simulink model "MainNew"  (R2021b)
settings: Solver=VariableStepAuto  StartTime=0.0  StopTime=10.0  RelTol=1e-3
undefined symbols (not defined in the file): c_Fuel, CM_FUEL_b, cmFuel_cmL, k_Fuel, L_TV, m_dot, m_iFuel, VRfromNED_cordT, W_LANDER
libraries: matrix_library x3, slpidlib x1, dspsrcs4 x1, shared6dof x1, aerolibanim x1, vrlib x1
settings Model: Creator=josepfamador  LastModifiedBy=josepfamador

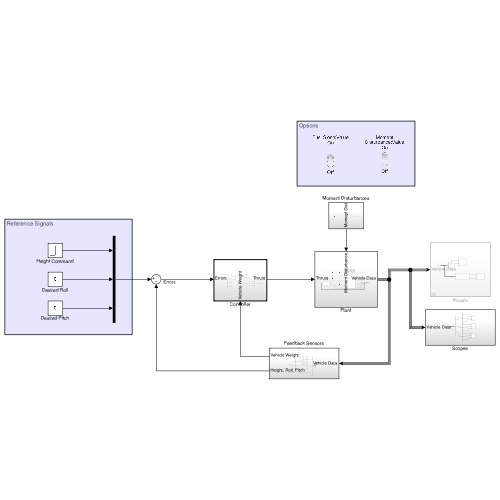
[thumbnail: Simulink's stored preview of the top-level diagram]
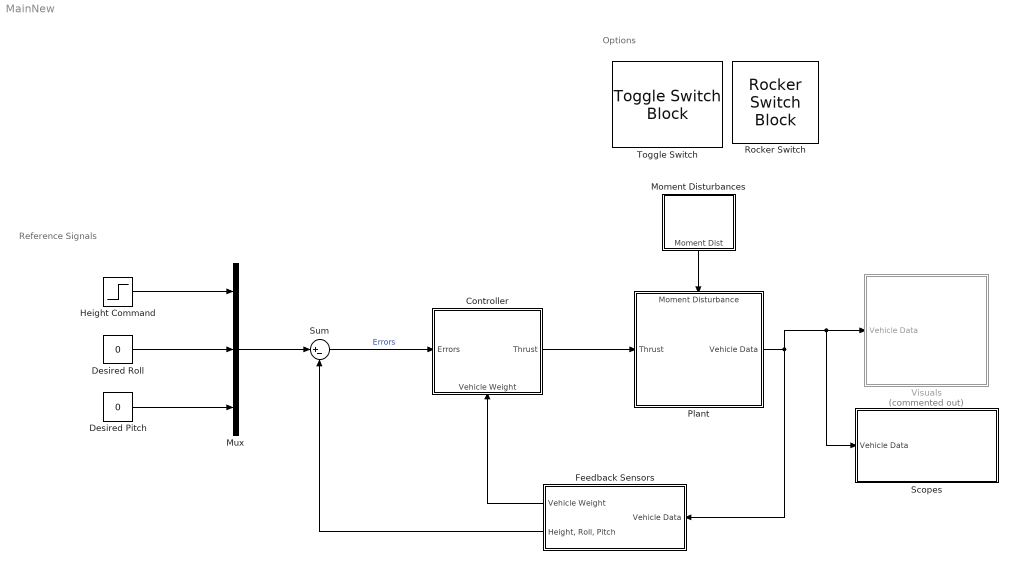
== system MainNew ==
  note: Options
  note: Reference Signals
  Controller : Subsystem  TreatAsAtomicUnit=on
      settings: PortSchema="{\"entries\":[{\"content\":{\"sides\":[{\"content\":{\"connectorIds\":[\"In1\"]},\"type\":\"ConnectorPlacement.EquallySpacedRectSide\",\"uuid\":\"a9e81047-82e7-465f-ace1-8f718b90561e\"},{\"content\":{\"connectorIds\":[\"Out1\"],\"side\":\"RIGHT\"},\"type\":\"ConnectorPlacement.EquallySpacedRectSide\",\"uuid\":\"e48627af-c2aa-4531-b804-41f44ff16765\"},{\"content\":{\"connectorIds\":[],\"side\":\"TOP\"},\"type\":\"ConnectorPlacement.EquallySpacedRectSide\",\"uuid\":\"f9e16229-b89b-4f8f-8331-a0f549979ea4\"},{\"content\":{\"connectorIds\":[\"In2\"],\"side\":\"BOTTOM\"},\"type\":\"ConnectorPlacement.EquallySpacedRectSide\",\"uuid\":\"04cdfde2-d4f0-49a2-8a73-ed462fcd7361\"}]},\"type\":\"ConnectorPlacement.EquallySpacedConnector\",\"uuid\":\"554d82b7-b70e-4d8b-909f-79f77f042d74\"}],\"packageUris\":[\"http://schema.mathworks.com/mf0/Connector/R2020b\"],\"version\":\"1.0\"}"
  Desired Pitch : Constant  Value=0
  Desired Roll : Constant  Value=0
  Feedback Sensors : Subsystem
  Height Command : Step  SampleTime=0
  Moment Disturbances : Subsystem
  Mux : Mux  Inputs=3
  Plant : Subsystem
      settings: PortSchema="{\"entries\":[{\"content\":{\"sides\":[{\"content\":{\"connectorIds\":[\"In1\"]},\"type\":\"ConnectorPlacement.EquallySpacedRectSide\",\"uuid\":\"a9e81047-82e7-465f-ace1-8f718b90561e\"},{\"content\":{\"connectorIds\":[\"Out1\"],\"side\":\"RIGHT\"},\"type\":\"ConnectorPlacement.EquallySpacedRectSide\",\"uuid\":\"e48627af-c2aa-4531-b804-41f44ff16765\"},{\"content\":{\"connectorIds\":[\"In2\"],\"side\":\"TOP\"},\"type\":\"ConnectorPlacement.EquallySpacedRectSide\",\"uuid\":\"f9e16229-b89b-4f8f-8331-a0f549979ea4\"}]},\"type\":\"ConnectorPlacement.EquallySpacedConnector\",\"uuid\":\"554d82b7-b70e-4d8b-909f-79f77f042d74\"}],\"packageUris\":[\"http://schema.mathworks.com/mf0/Connector/R2020b\"],\"version\":\"1.0\"}"
  Rocker Switch : RockerSwitchBlock
      settings: Values={{'Off', 'On'}, [0 1]}
  Scopes : Subsystem
  Sum : Sum  Inputs=|+-
  Toggle Switch : ToggleSwitchBlock
      settings: Values={{'Off', 'On'}, [0 1]}
  Visuals : Subsystem  Commented=on
  wires:
  Moment Disturbances/1(Moment Dist) -> Plant/2(Moment Disturbance)
  Plant/1(Vehicle Data) -> Feedback Sensors/1(Vehicle Data), Scopes/1(Vehicle Data), Visuals/1(Vehicle Data)
  Desired Pitch/1 -> Mux/3
  Desired Roll/1 -> Mux/2
  Height Command/1 -> Mux/1
  Mux/1 -> Sum/1
  Feedback Sensors/2("Height, Roll, Pitch") -> Sum/2
  Sum/1 -> Controller/1(Errors)  "Errors"
  Controller/1(Thrust) -> Plant/1(Thrust)
  Feedback Sensors/1(Vehicle Weight) -> Controller/2(Vehicle Weight)

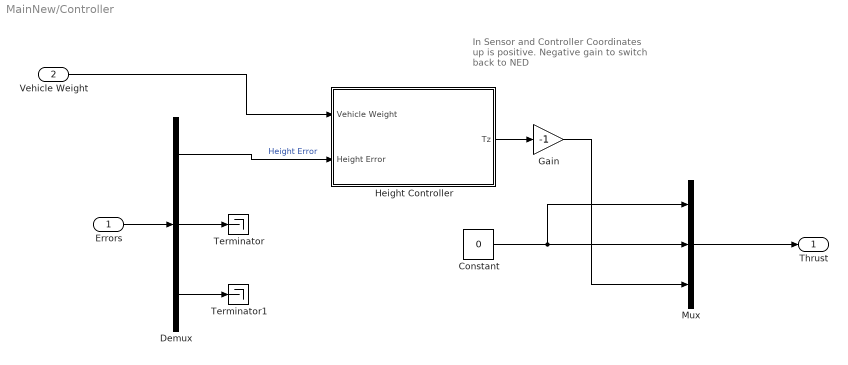
== system MainNew/Controller ==
  note: In Sensor and Controller Coordinates up is positive. Negative gain to switch back to NED
  Errors : Inport
  Vehicle Weight : Inport  Port=2
  Constant : Constant  Value=0
  Demux : Demux  Outputs=3
  Gain : Gain  Gain=-1
  Height Controller : Subsystem
  Mux : Mux  Inputs=3
  Terminator : Terminator
  Terminator1 : Terminator
  Thrust : Outport
  wires:
  Errors/1 -> Demux/1
  Demux/1 -> Height Controller/2(Height Error)  "Height Error"
  Vehicle Weight/1 -> Height Controller/1(Vehicle Weight)
  Mux/1 -> Thrust/1
  Height Controller/1(Tz) -> Gain/1
  Constant/1 -> Mux/2, Mux/1
  Demux/2 -> Terminator/1
  Demux/3 -> Terminator1/1
  Gain/1 -> Mux/3

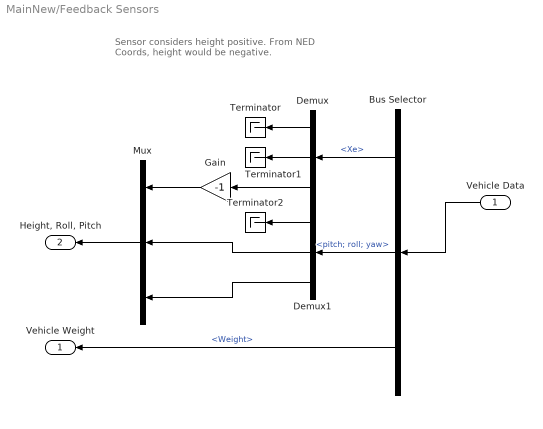
== system MainNew/Feedback Sensors ==
  note: Sensor considers height positive.
      | From NED Coords, height would be negative.
  Vehicle Data : Inport
  Bus Selector : BusSelector  OutputSignals=Xe,pitch; roll; yaw,Weight
  Demux : Demux  Outputs=3
  Demux1 : Demux  Outputs=3
  Gain : Gain  Gain=-1
  Mux : Mux  Inputs=3
  Terminator : Terminator
  Terminator1 : Terminator
  Terminator2 : Terminator
  Vehicle Weight : Outport
  "Height, Roll, Pitch" : Outport  Port=2
  wires:
  Vehicle Data/1 -> Bus Selector/1
  Bus Selector/1 -> Demux/1  "<Xe>"
  Bus Selector/2 -> Demux1/1  "<pitch; roll; yaw>"
  Demux/3 -> Gain/1
  Demux1/2 -> Mux/2
  Demux1/3 -> Mux/3
  Demux/1 -> Terminator/1
  Demux/2 -> Terminator1/1
  Demux1/1 -> Terminator2/1
  Mux/1 -> "Height, Roll, Pitch"/1
  Gain/1 -> Mux/1
  Bus Selector/3 -> Vehicle Weight/1  "<Weight>"

== system MainNew/Moment Disturbances ==
  Disturbance Vector : Subsystem
  Moment Disturbance : Constant  Value=0
  Slider : SliderBlock  ScaleMax=20
  Moment Dist : Outport
  wires:
  Disturbance Vector/1(Out1) -> Moment Dist/1
  Moment Disturbance/1 -> Disturbance Vector/Enable

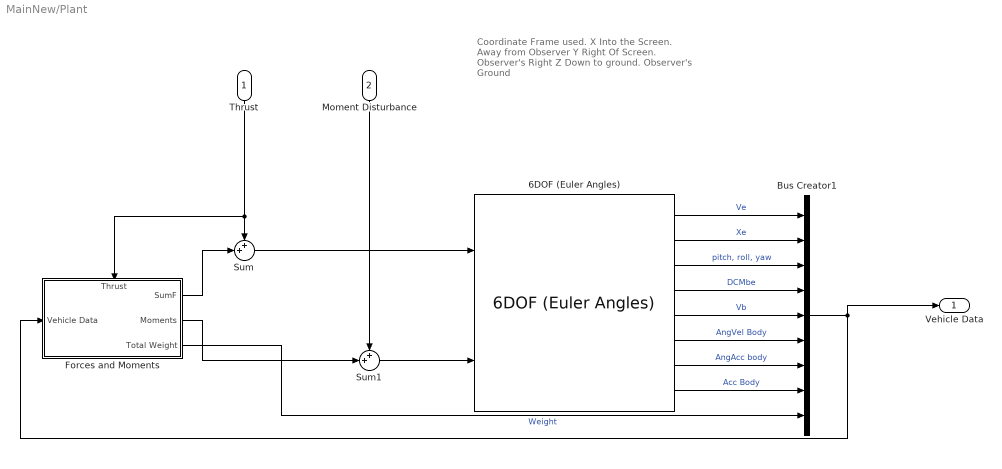
== system MainNew/Plant ==
  note: Coordinate Frame used.
      | X
      | Into the Screen. Away from Observer
      |
      | Y
      | Right Of Screen. Observer's Right
      |
      | Z
      | Down to ground. Observer's Ground
  Thrust : Inport
  Moment Disturbance : Inport  Port=2
  6DOF (Euler Angles) : shared6dof/6DOF (Euler Angles)  units=Metric (MKS)  mtype=Fixed  rep=Euler Angles  xme_0=[0 0 0]  Vm_0=[0 0 0]  eul_0=[0 0 0]  pm_0=[0 0 0]  mass_0=M_lander  mass_e=0.5  mass_f=2.0  inertia=I  inertia_e=eye(3)  inertia_f=2*eye(3)  k_quat=1.0  vre_flag=on  abi_flag=off  aMode=0  xme_statename=''  Vm_statename=''  eul_statename=''  quat_statename=''  pm_statename=''  mass_statename=''
      settings: SourceProductBaseCode=AE,PW,DR,MT,UV,VE
  Bus Creator1 : BusCreator  Inputs=9
  Forces and Moments : Subsystem
      settings: PortSchema="{\"entries\":[{\"content\":{\"sides\":[{\"content\":{\"connectorIds\":[\"In1\"]},\"type\":\"ConnectorPlacement.EquallySpacedRectSide\",\"uuid\":\"828f15e3-cbad-415f-85fb-ba6a8e0cd3b9\"},{\"content\":{\"connectorIds\":[\"Out1\",\"Out2\",\"Out3\"],\"side\":\"RIGHT\"},\"type\":\"ConnectorPlacement.EquallySpacedRectSide\",\"uuid\":\"5000816a-8e0b-4f65-bf77-7d05076903d9\"},{\"content\":{\"connectorIds\":[\"In2\"],\"side\":\"TOP\"},\"type\":\"ConnectorPlacement.EquallySpacedRectSide\",\"uuid\":\"57f53c13-0af9-4c97-9cf0-1ba4f356b699\"}]},\"type\":\"ConnectorPlacement.EquallySpacedConnector\",\"uuid\":\"7fdc047f-04f4-4b62-afef-380f9e9b929b\"}],\"packageUris\":[\"http://schema.mathworks.com/mf0/Connector/R2020b\"],\"version\":\"1.0\"}"
  Sum : Sum  Inputs=++|
  Sum1 : Sum  Inputs=++|
  Vehicle Data : Outport
  wires:
  6DOF (Euler Angles)/7 -> Bus Creator1/7  "AngAcc body"
  6DOF (Euler Angles)/3 -> Bus Creator1/3  "pitch, roll, yaw"
  Sum/1 -> 6DOF (Euler Angles)/1
  Thrust/1 -> Forces and Moments/2(Thrust), Sum/1
  6DOF (Euler Angles)/4 -> Bus Creator1/4  "DCMbe"
  Forces and Moments/1(SumF) -> Sum/2
  Forces and Moments/2(Moments) -> Sum1/2
  6DOF (Euler Angles)/6 -> Bus Creator1/6  "AngVel Body"
  6DOF (Euler Angles)/1 -> Bus Creator1/1  "Ve"
  6DOF (Euler Angles)/2 -> Bus Creator1/2  "Xe"
  6DOF (Euler Angles)/5 -> Bus Creator1/5  "Vb"
  6DOF (Euler Angles)/8 -> Bus Creator1/8  "Acc Body"
  Bus Creator1/1 -> Vehicle Data/1, Forces and Moments/1(Vehicle Data)
  Sum1/1 -> 6DOF (Euler Angles)/2
  Moment Disturbance/1 -> Sum1/1
  Forces and Moments/3(Total Weight) -> Bus Creator1/9  "Weight"

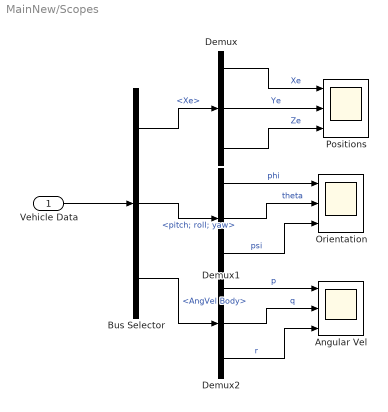
== system MainNew/Scopes ==
  Vehicle Data : Inport
  Angular Vel : Scope  NumInputPorts=3
  Bus Selector : BusSelector  OutputSignals=Xe,pitch; roll; yaw,AngVel Body
  Demux : Demux  Outputs=3
  Demux1 : Demux  Outputs=3
  Demux2 : Demux  Outputs=3
  Orientation : Scope  NumInputPorts=3
  Positions : Scope  NumInputPorts=3
  wires:
  Vehicle Data/1 -> Bus Selector/1
  Bus Selector/1 -> Demux/1  "<Xe>"
  Bus Selector/3 -> Demux2/1  "<AngVel Body>"
  Bus Selector/2 -> Demux1/1  "<pitch; roll; yaw>"
  Demux/2 -> Positions/2  "Ye"
  Demux/1 -> Positions/1  "Xe"
  Demux/3 -> Positions/3  "Ze"
  Demux1/1 -> Orientation/1  "phi"
  Demux1/2 -> Orientation/2  "theta"
  Demux1/3 -> Orientation/3  "psi"
  Demux2/2 -> Angular Vel/2  "q"
  Demux2/1 -> Angular Vel/1  "p"
  Demux2/3 -> Angular Vel/3  "r"

== system MainNew/Visuals ==
  Vehicle Data : Inport
  6DoF Animation1 : aerolibanim/6DoF Animation  u1=[-5 5 -5 5 0 4]  u2=0.1  u3=1  u4=[0 0 -1]  u5=Fixed position  u6=[-10 0 0]  u7=45  u8=off
  Bus Selector : BusSelector  OutputSignals=Xe,pitch; roll; yaw
  Coordinate Transforms : Subsystem
  VR Sink : vrlib/VR Sink  InstantiateOnLoad=on  SampleTime=0.1  ViewEnable=on  RemoteChange=off  RemoteView=off  FieldsWritten=Lander.rotation.4.1.1.double#Lander.translation.3.1.1.double  WorldFileName=/Users/josepfamador/RPL_controls/vrsinkstuff/V6b.x3d  AutoView=off  VideoDimensions=[]  AllowVariableSize=off
  wires:
  Bus Selector/1 -> 6DoF Animation1/1  "<Xe>"
  Bus Selector/2 -> 6DoF Animation1/2  "<pitch; roll; yaw>"
  Vehicle Data/1 -> Bus Selector/1, Coordinate Transforms/1(Vehicle Data)
  Coordinate Transforms/1(VR Rotation) -> VR Sink/1
  Coordinate Transforms/2(VR Translation) -> VR Sink/2

== system MainNew/Controller/Height Controller ==
  Vehicle Weight : Inport
  Height Error : Inport  Port=2
  Dot Product : DotProduct  InputSameDT=on  OutDataTypeStr=Inherit: Inherit via internal rule
  PID Controller : slpidlib/PID Controller  Controller=PID  Form=Parallel  TimeDomain=Continuous-time  UseExternalTs=off  SampleTime=-1  IntegratorMethod=Forward Euler  FilterMethod=Forward Euler  ControllerParametersSource=internal  P=0.203941393902336  I=0.000548507911387826  D=13.3428538970744  UseFilter=on  N=45.4968011971303  TunerSelectOption=Transfer Function Based (PID Tuner App)  InitialConditionSource=internal  InitialConditionForIntegrator=0  InitialConditionForFilter=0  DifferentiatorICPrevScaledInput=0  ExternalReset=none  TrackingMode=off  Kt=1  LimitOutput=off  SatLimitsSource=internal  UpperSaturationLimit=inf  LowerSaturationLimit=-inf  LinearizeAsGain=on  AntiWindupMode=none  Kb=1  POutMin=[]  POutMax=[]  IOutMin=[]  IOutMax=[]  DOutMin=[]  DOutMax=[]  NOutMin=[]  NOutMax=[]  SumOutMin=[]  SumOutMax=[]  SaturationOutMin=[]  SaturationOutMax=[]  PParamMin=[]  PParamMax=[]  IParamMin=[]  IParamMax=[]  DParamMin=[]  DParamMax=[]  NParamMin=[]  NParamMax=[]  KbParamMin=[]  KbParamMax=[]  KtParamMin=[]  KtParamMax=[]  KbOutMin=[]  KbOutMax=[]  KtOutMin=[]  KtOutMax=[]  IntegratorOutMin=[]  IntegratorOutMax=[]  FilterOutMin=[]  FilterOutMax=[]  SumI1OutMin=[]  SumI1OutMax=[]  SumI2OutMin=[]  SumI2OutMax=[]  SumI3OutMin=[]  SumI3OutMax=[]  SumI4OutMin=[]  SumI4OutMax=[]  SumDOutMin=[]  SumDOutMax=[]  DifferentiatorOutMin=[]  DifferentiatorOutMax=[]  FilterDiffOutCoefMin=[]  FilterDiffOutCoefMax=[]  ReciprocalOutMin=[]  ReciprocalOutMax=[]  SumDenOutMin=[]  SumDenOutMax=[]  SumNumOutMin=[]  SumNumOutMax=[]  DivideOutMin=[]  DivideOutMax=[]  UdiffTsProdOutMin=[]  UdiffTsProdOutMax=[]  NTsProdOutMin=[]  NTsProdOutMax=[]  UintegralTsProdOutMin=[]  UintegralTsProdOutMax=[]  UngainTsProdOutMin=[]  UngainTsProdOutMax=[]  IntegratorContinuousStateAttributes=''  IntegratorStateMustResolveToSignalObject=off  IntegratorRTWStateStorageClass=Auto  FilterContinuousStateAttributes=''  FilterStateMustResolveToSignalObject=off  FilterRTWStateStorageClass=Auto  ParallelPVariant=InternalParameters  IdealPVariant=Disabled  IVariant=InternalParameters  DVariant=InternalParameters  IntegratorVariant=Continuous  SatVariant=Disabled  AWVariant=Passthrough  PCopyVariant=Disabled  TRVariant=Disabled  FdbkBlocksVariant=Forward  IdealPFdbkVariant=Disabled  SatFdbkVariant=Disabled  DerivativeFilterVariant=ContFilter  NVariant=InternalParameters  NCopyVariant=Disabled  FilterICVariant=InternalICsFilter  IntegratorICVariant=InternalICs  ExternalResetVariant=Disabled  TRSumVariant=Passthrough  SumFdbkVariant=Disabled  SumVariant=Sum_PID  TsampFilterVariant=InternalTs  TsampNgainVariant=Passthrough  TsampIntegralVariant=Passthrough  ExternalSaturationOutDataTypeStr=Inherit: Same as second input
  Square Root : Sqrt  SaturateOnIntegerOverflow=on
  Sum : Sum  Inputs=++|
  Tz : Outport
  wires:
  Height Error/1 -> PID Controller/1
  Vehicle Weight/1 -> Dot Product/1, Dot Product/2
  Dot Product/1 -> Square Root/1
  PID Controller/1 -> Sum/2  "Thrust Difference"
  Square Root/1 -> Sum/1
  Sum/1 -> Tz/1

== system MainNew/Moment Disturbances/Disturbance Vector ==
  Enable : EnablePort
  Constant : Constant  Value=0
  Discrete Impulse : dspsrcs4/Discrete  Impulse  Delay=0  SampleTime=1  FrameSample=1  OutputFrames=off  dataType=double  isSigned=on  wordLen=16  udDataType=sfix(16)  fracBitsMode=Best precision  numFracBits=15  OutDataTypeStr=double  LastOutDataTypeStr=double
  Impulse Magnitude (Newtons) : Gain  Gain=0.3610372340425532
  Mux : Mux  Inputs=3
  Out1 : Outport
  wires:
  Mux/1 -> Out1/1
  Impulse Magnitude (Newtons)/1 -> Mux/2
  Discrete Impulse/1 -> Impulse Magnitude (Newtons)/1
  Constant/1 -> Mux/3, Mux/1

== system MainNew/Plant/Forces and Moments ==
  Vehicle Data : Inport
  Thrust : Inport  Port=2
  Forces Body Fixed Frame : Subsystem  TreatAsAtomicUnit=on
      settings: PortSchema="{\"entries\":[{\"content\":{\"sides\":[{\"content\":{\"connectorIds\":[\"In1\"]},\"type\":\"ConnectorPlacement.EquallySpacedRectSide\",\"uuid\":\"828f15e3-cbad-415f-85fb-ba6a8e0cd3b9\"},{\"content\":{\"connectorIds\":[\"Out1\",\"Out2\"],\"side\":\"RIGHT\"},\"type\":\"ConnectorPlacement.EquallySpacedRectSide\",\"uuid\":\"5000816a-8e0b-4f65-bf77-7d05076903d9\"},{\"content\":{\"connectorIds\":[],\"side\":\"TOP\"},\"type\":\"ConnectorPlacement.EquallySpacedRectSide\",\"uuid\":\"57f53c13-0af9-4c97-9cf0-1ba4f356b699\"},{\"content\":{\"connectorIds\":[\"Out3\",\"Out4\"],\"side\":\"BOTTOM\"},\"type\":\"ConnectorPlacement.EquallySpacedRectSide\",\"uuid\":\"07d00598-10e4-47df-ac26-33e6f3a9eead\"}]},\"type\":\"ConnectorPlacement.EquallySpacedConnector\",\"uuid\":\"7fdc047f-04f4-4b62-afef-380f9e9b929b\"}],\"packageUris\":[\"http://schema.mathworks.com/mf0/Connector/R2020b\"],\"version\":\"1.0\"}"
  Moments Body Fixed : Subsystem
      settings: PortSchema="{\"entries\":[{\"content\":{\"sides\":[{\"content\":{\"connectorIds\":[\"In1\"]},\"type\":\"ConnectorPlacement.EquallySpacedRectSide\",\"uuid\":\"bf632890-9061-4ebf-b839-17051433f7d2\"},{\"content\":{\"connectorIds\":[\"Out1\"],\"side\":\"RIGHT\"},\"type\":\"ConnectorPlacement.EquallySpacedRectSide\",\"uuid\":\"d3255547-983f-46fe-8ffa-de3f6c331a2a\"},{\"content\":{\"connectorIds\":[\"In2\",\"In3\"],\"side\":\"TOP\"},\"type\":\"ConnectorPlacement.EquallySpacedRectSide\",\"uuid\":\"18f3806f-6d56-407f-aadd-d25baf8c86b7\"}]},\"type\":\"ConnectorPlacement.EquallySpacedConnector\",\"uuid\":\"1b0eb8e4-97ea-4203-914f-8b852a07c841\"}],\"packageUris\":[\"http://schema.mathworks.com/mf0/Connector/R2020b\"],\"version\":\"1.0\"}"
  SumF : Outport
  Moments : Outport  Port=2
  Total Weight : Outport  Port=3
  wires:
  Forces Body Fixed Frame/1(SumF) -> SumF/1
  Moments Body Fixed/1(Moment) -> Moments/1
  Forces Body Fixed Frame/3(Fuel Slosh Vector) -> Moments Body Fixed/2(Slosh)
  Thrust/1 -> Moments Body Fixed/1(Thrust)
  Forces Body Fixed Frame/4(Weight Fuel (Body Fixed)) -> Moments Body Fixed/3(Weight Body Fixed)
  Vehicle Data/1 -> Forces Body Fixed Frame/1(Vehicle Data)
  Forces Body Fixed Frame/2(Total Weight) -> Total Weight/1

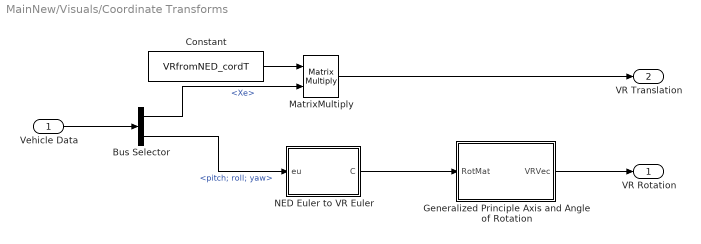
== system MainNew/Visuals/Coordinate Transforms ==
  Vehicle Data : Inport
  Bus Selector : BusSelector  OutputSignals=Xe,pitch; roll; yaw
  Constant : Constant  Value=VRfromNED_cordT
  Generalized Principle Axis and Angle of Rotation : MATLAB Function  TreatAsAtomicUnit=on
  MatrixMultiply : Product  Multiplication=Matrix(*)
  NED Euler to VR Euler : MATLAB Function  TreatAsAtomicUnit=on
  VR Rotation : Outport
  VR Translation : Outport  Port=2
  wires:
  Vehicle Data/1 -> Bus Selector/1
  Constant/1 -> MatrixMultiply/1
  Bus Selector/1 -> MatrixMultiply/2  "<Xe>"
  Bus Selector/2 -> NED Euler to VR Euler/1(eu)  "<pitch; roll; yaw>"
  NED Euler to VR Euler/1(C) -> Generalized Principle Axis and Angle of Rotation/1(RotMat)
  MatrixMultiply/1 -> VR Translation/1
  Generalized Principle Axis and Angle of Rotation/1(VRVec) -> VR Rotation/1

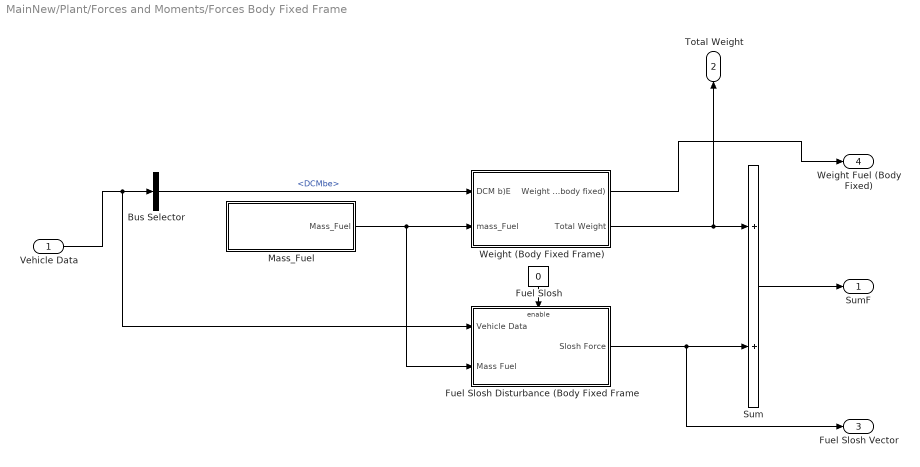
== system MainNew/Plant/Forces and Moments/Forces Body Fixed Frame ==
  Vehicle Data : Inport
  Bus Selector : BusSelector  OutputSignals=DCMbe
  Fuel Slosh : Constant  Value=0
  Fuel Slosh Disturbance (Body Fixed Frame : Subsystem
  Mass_Fuel : Subsystem
  Sum : Sum
  Weight (Body Fixed Frame) : Subsystem
  SumF : Outport
  Total Weight : Outport  Port=2
  Fuel Slosh Vector : Outport  Port=3
  Weight Fuel (Body Fixed) : Outport  Port=4
  wires:
  Mass_Fuel/1(Mass_Fuel) -> Fuel Slosh Disturbance (Body Fixed Frame/2(Mass Fuel), Weight (Body Fixed Frame)/2(mass_Fuel)
  Weight (Body Fixed Frame)/2(Total Weight) -> Total Weight/1, Sum/1
  Fuel Slosh Disturbance (Body Fixed Frame/1(Slosh Force) -> Fuel Slosh Vector/1, Sum/2
  Sum/1 -> SumF/1
  Fuel Slosh/1 -> Fuel Slosh Disturbance (Body Fixed Frame/Enable
  Weight (Body Fixed Frame)/1(Weight Fuel (body fixed)) -> Weight Fuel (Body Fixed)/1
  Vehicle Data/1 -> Fuel Slosh Disturbance (Body Fixed Frame/1(Vehicle Data), Bus Selector/1
  Bus Selector/1 -> Weight (Body Fixed Frame)/1(DCM b)E)  "<DCMbe>"

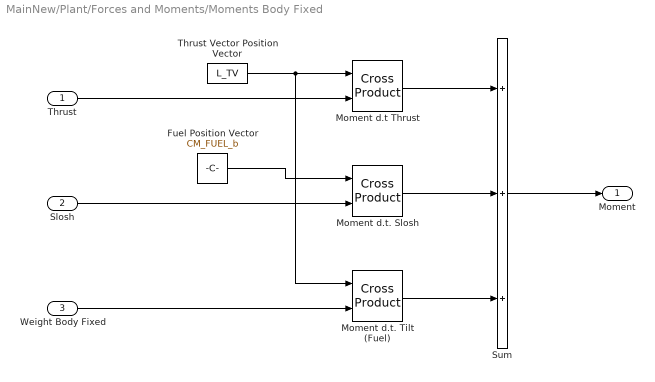
== system MainNew/Plant/Forces and Moments/Moments Body Fixed ==
  Thrust : Inport
  Slosh : Inport  Port=2
  Weight Body Fixed : Inport  Port=3
  Fuel Position Vector : Constant  Value=CM_FUEL_b
  Moment d.t Thrust : matrix_library/Cross Product
      settings: SourceProductBaseCode=SL
  Moment d.t. Slosh : matrix_library/Cross Product
      settings: SourceProductBaseCode=SL
  Moment d.t. Tilt (Fuel) : matrix_library/Cross Product
      settings: SourceProductBaseCode=SL
  Sum : Sum  Inputs=+++
  Thrust Vector Position Vector : Constant  Value=L_TV
  Moment : Outport
  wires:
  Thrust/1 -> Moment d.t Thrust/2
  Thrust Vector Position Vector/1 -> Moment d.t. Tilt (Fuel)/1, Moment d.t Thrust/1
  Slosh/1 -> Moment d.t. Slosh/2
  Fuel Position Vector/1 -> Moment d.t. Slosh/1
  Weight Body Fixed/1 -> Moment d.t. Tilt (Fuel)/2
  Moment d.t. Tilt (Fuel)/1 -> Sum/3
  Moment d.t. Slosh/1 -> Sum/2
  Moment d.t Thrust/1 -> Sum/1
  Sum/1 -> Moment/1

== system MainNew/Plant/Forces and Moments/Forces Body Fixed Frame/Fuel Slosh Disturbance (Body Fixed Frame ==
  note: 0 Disturbance in Z Body fixed Frame From Fuel Slosh
  Vehicle Data : Inport
  Mass Fuel : Inport  Port=2
  Enable : EnablePort
  Constant : Constant  Value=0
  Forces Slosh : Subsystem
  Mux : Mux  Inputs=3
  Subsystem : Subsystem
  Slosh Force : Outport
  wires:
  Subsystem/1("phi, phi_d, phi_dd") -> Forces Slosh/1("EA, EAd, EAdd")
  Subsystem/2("theta, theta_d, theta_dd") -> Forces Slosh/2("EA, EAd, EAdd1")
  Mass Fuel/1 -> Forces Slosh/3(Mass Fuel)
  Constant/1 -> Mux/3
  Forces Slosh/1(Fx) -> Mux/1
  Forces Slosh/2(Fy) -> Mux/2
  Mux/1 -> Slosh Force/1
  Vehicle Data/1 -> Subsystem/1(Vehicle Data)

== system MainNew/Plant/Forces and Moments/Forces Body Fixed Frame/Mass_Fuel ==
  note: m_dot set to 0
  Clock : Clock
  Sum : Sum  Inputs=+-|
  mass_burn_rate : Gain  Gain=m_dot
  mass_intial_fuel : Constant  Value=m_iFuel
  Mass_Fuel : Outport
  wires:
  mass_burn_rate/1 -> Sum/2
  Sum/1 -> Mass_Fuel/1
  mass_intial_fuel/1 -> Sum/1
  Clock/1 -> mass_burn_rate/1

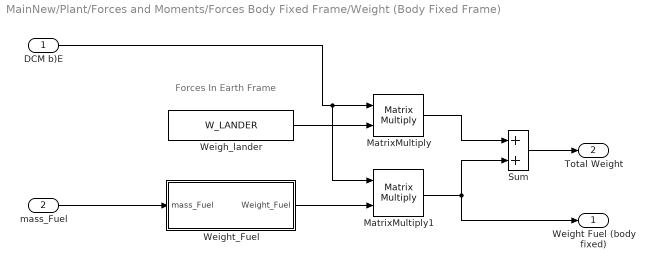
== system MainNew/Plant/Forces and Moments/Forces Body Fixed Frame/Weight (Body Fixed Frame) ==
  note: Forces In Earth Frame
  DCM b)E : Inport
  mass_Fuel : Inport  Port=2
  MatrixMultiply : Product  Multiplication=Matrix(*)
  MatrixMultiply1 : Product  Multiplication=Matrix(*)
  Sum : Sum
  Weigh_lander : Constant  Value=W_LANDER
  Weight_Fuel : Subsystem  TreatAsAtomicUnit=on
  Weight Fuel (body fixed) : Outport
  Total Weight : Outport  Port=2
  wires:
  mass_Fuel/1 -> Weight_Fuel/1(mass_Fuel)
  DCM b)E/1 -> MatrixMultiply1/1, MatrixMultiply/1
  MatrixMultiply1/1 -> Weight Fuel (body fixed)/1, Sum/2
  MatrixMultiply/1 -> Sum/1
  Weight_Fuel/1(Weight_Fuel) -> MatrixMultiply1/2
  Weigh_lander/1 -> MatrixMultiply/2
  Sum/1 -> Total Weight/1

== system MainNew/Plant/Forces and Moments/Forces Body Fixed Frame/Fuel Slosh Disturbance (Body Fixed Frame/Forces Slosh ==
  "EA, EAd, EAdd" : Inport
  "EA, EAd, EAdd1" : Inport  Port=2
  Mass Fuel : Inport  Port=3
  Constant : Constant  Value=cmFuel_cmL
  Subsystem1 : Subsystem
  Subsystem2 : Subsystem
  Fx : Outport
  Fy : Outport  Port=2
  wires:
  "EA, EAd, EAdd1"/1 -> Subsystem2/1("EA, EAd, EAdd")  "Pitch"
  Subsystem2/1(Fy) -> Fy/1
  "EA, EAd, EAdd"/1 -> Subsystem1/1("EA, EAd, EAdd")  "Roll"
  Subsystem1/1(Fx) -> Fx/1
  Constant/1 -> Subsystem2/3(Arm Length), Subsystem1/3(Arm Length)
  Mass Fuel/1 -> Subsystem1/2(Mass Fuel), Subsystem2/2(Mass Fuel)

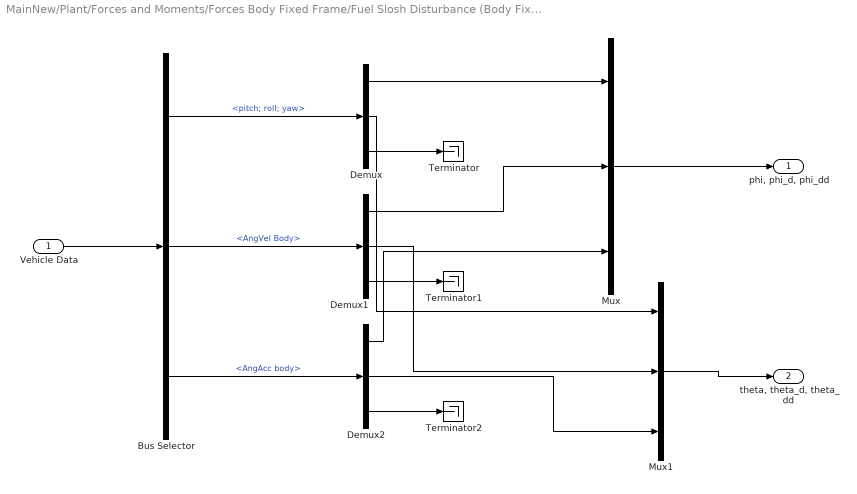
== system MainNew/Plant/Forces and Moments/Forces Body Fixed Frame/Fuel Slosh Disturbance (Body Fixed Frame/Subsystem ==
  Vehicle Data : Inport
  Bus Selector : BusSelector  OutputSignals=pitch; roll; yaw,AngVel Body,AngAcc body
  Demux : Demux  Outputs=3
  Demux1 : Demux  Outputs=3
  Demux2 : Demux  Outputs=3
  Mux : Mux  Inputs=3
  Mux1 : Mux  Inputs=3
  Terminator : Terminator
  Terminator1 : Terminator
  Terminator2 : Terminator
  "phi, phi_d, phi_dd" : Outport
  "theta, theta_d, theta_dd" : Outport  Port=2
  wires:
  Bus Selector/1 -> Demux/1  "<pitch; roll; yaw>"
  Bus Selector/2 -> Demux1/1  "<AngVel Body>"
  Bus Selector/3 -> Demux2/1  "<AngAcc body>"
  Demux/1 -> Mux/1
  Demux1/1 -> Mux/2
  Demux2/1 -> Mux/3
  Mux/1 -> "phi, phi_d, phi_dd"/1
  Demux/2 -> Mux1/1
  Demux1/2 -> Mux1/2
  Demux2/2 -> Mux1/3
  Demux/3 -> Terminator/1
  Demux1/3 -> Terminator1/1
  Demux2/3 -> Terminator2/1
  Mux1/1 -> "theta, theta_d, theta_dd"/1
  Vehicle Data/1 -> Bus Selector/1

== system MainNew/Plant/Forces and Moments/Forces Body Fixed Frame/Weight (Body Fixed Frame)/Weight_Fuel ==
  mass_Fuel : Inport
  Constant : Constant  Value=0
  Mux : Mux  Inputs=3
  Weight_Fuel : Outport
  wires:
  Constant/1 -> Mux/2, Mux/1
  mass_Fuel/1 -> Mux/3
  Mux/1 -> Weight_Fuel/1

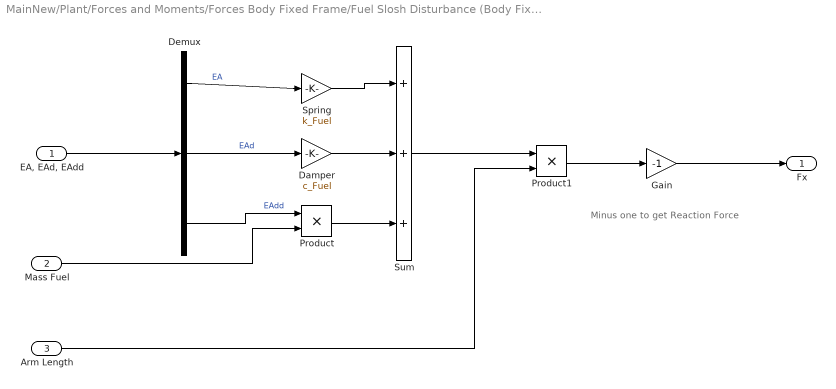
== system MainNew/Plant/Forces and Moments/Forces Body Fixed Frame/Fuel Slosh Disturbance (Body Fixed Frame/Forces Slosh/Subsystem1 ==
  note: Minus one to get Reaction Force
  "EA, EAd, EAdd" : Inport
  Mass Fuel : Inport  Port=2
  Arm Length : Inport  Port=3
  Damper : Gain  Gain=c_Fuel
  Demux : Demux  Outputs=3
  Gain : Gain  Gain=-1
  Product : Product
  Product1 : Product
  Spring : Gain  Gain=k_Fuel
  Sum : Sum  Inputs=+++
  Fx : Outport
  wires:
  Demux/1 -> Spring/1  "EA"
  Demux/2 -> Damper/1  "EAd"
  Demux/3 -> Product/1  "EAdd"
  Mass Fuel/1 -> Product/2
  Product/1 -> Sum/3
  Damper/1 -> Sum/2
  Spring/1 -> Sum/1
  "EA, EAd, EAdd"/1 -> Demux/1
  Sum/1 -> Product1/1
  Arm Length/1 -> Product1/2
  Product1/1 -> Gain/1
  Gain/1 -> Fx/1

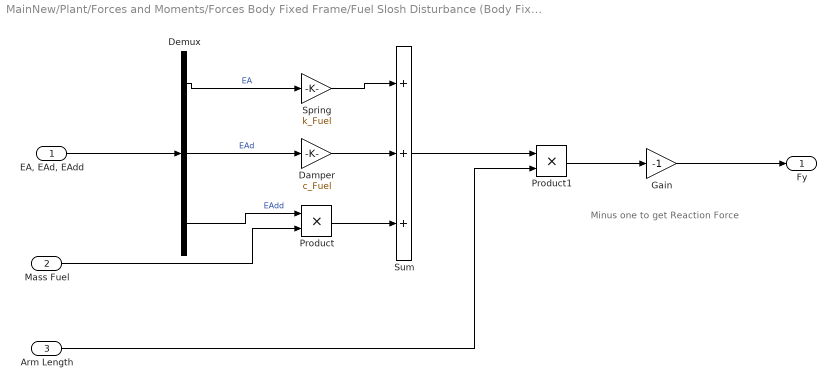
== system MainNew/Plant/Forces and Moments/Forces Body Fixed Frame/Fuel Slosh Disturbance (Body Fixed Frame/Forces Slosh/Subsystem2 ==
  note: Minus one to get Reaction Force
  "EA, EAd, EAdd" : Inport
  Mass Fuel : Inport  Port=2
  Arm Length : Inport  Port=3
  Damper : Gain  Gain=c_Fuel
  Demux : Demux  Outputs=3
  Gain : Gain  Gain=-1
  Product : Product
  Product1 : Product
  Spring : Gain  Gain=k_Fuel
  Sum : Sum  Inputs=+++
  Fy : Outport
  wires:
  Demux/1 -> Spring/1  "EA"
  Demux/2 -> Damper/1  "EAd"
  Demux/3 -> Product/1  "EAdd"
  Mass Fuel/1 -> Product/2
  Product/1 -> Sum/3
  Damper/1 -> Sum/2
  Spring/1 -> Sum/1
  "EA, EAd, EAdd"/1 -> Demux/1
  Sum/1 -> Product1/1
  Arm Length/1 -> Product1/2
  Product1/1 -> Gain/1
  Gain/1 -> Fy/1

== matlab function MainNew/Visuals/Coordinate Transforms/Generalized Principle Axis and Angle of Rotation ==
  data: VRVec output; RotMat input
function VRVec  = fcn(RotMat)
% Rotation algorithms obtained form "Spacecraft Dynamics & Control (ARO
% 4090 text) pg 21 
phi = acos((trace(RotMat) -  1)/2); % eq 1.27
A = 1/(sin(phi)) * [RotMat(2,3) - RotMat(3,2)
                    RotMat(3,1) - RotMat(1,3)
                    RotMat(1,2) - RotMat(2,1)]; % eq 1.28
VRVec = [A;phi];

== matlab function MainNew/Visuals/Coordinate Transforms/NED Euler to VR Euler ==
  data: eu input; C output
function C = fcn(eu)
psi = eu(1); % FIrst rotation about NEDbody Fixed x
theta = eu(2); % Second rot about NEd Body fixed y
phi = eu(3); % Second rotation about NedBody Fixed Z

alpha =  -psi; % First rot about VR Body Fixed
beta = theta; % Second rotation about VR Body Fixed
gamm = -phi; % Thirst rot about VR Body fixed
 
Cz = [cos(alpha)  sin(alpha) 0
      -sin(alpha) cos(alpha) 0
      0           0          1];
Cx = [1 0         0
      0 cos(beta)  sin(beta)
      0 -sin(beta) cos(beta)];
Cy = [cos(gamm) 0 -sin(gamm)
      0         1 0
      sin(gamm) 0 cos(gamm)];
C = Cy * Cx * Cz;
